simulink model "simulazione_completa"  (R2020a)
settings: Solver=VariableStepAuto  StartTime=0.0  StopTime=1.1*Ts*p  RelTol=1e-3
values from neighbouring files (symbols this model uses):
  A = A_lin_eq    [Ascensione.m]    (also in Sistema.m; f_tilde.m = [-0.0014   -0.0000         0)
  Ad = sysD.a    [Ascensione.m]    (also in Sistema.m)
  B = B_lin_eq(:,1)    [Ascensione.m]    (also in Sistema.m; f_tilde.m = [0.0014)
  Bd = sysD.b    [Ascensione.m]    (also in Sistema.m)
  C = [0 1 0]    [Ascensione.m]    (also in Sistema.m)
  p = 1000    [Pianificazione_senza_vincoli.m]    (also in Pianificazione_vincoli_ingresso.m = p+1; Pianificazione_vincoli_stato.m = ceil(p*1.1); tpr.m = p0*(1-L/T0*z)^(g/(R*L)))
  reg = ss(A+B*K+L*C,-L,-K,0)    [Ascensione.m]    (also in Sistema.m)
  Ts = 0.05    [Ascensione.m]    (also in Sistema.m)
  Vlim = -double(sqrt(2*subs(m,[x1,x2],[x1_eq,x2_eq])*g/rho_bar/Sz/Cz))    [Sistema.m]
  x_0 = [0 0 0].'    [Pianificazione_senza_vincoli.m]
settings Model: Creator=andre  LastModifiedBy=andre
settings OptimizationCC: BlockReduction=off  DefaultParameterBehavior=Inlined  BufferReuse=off

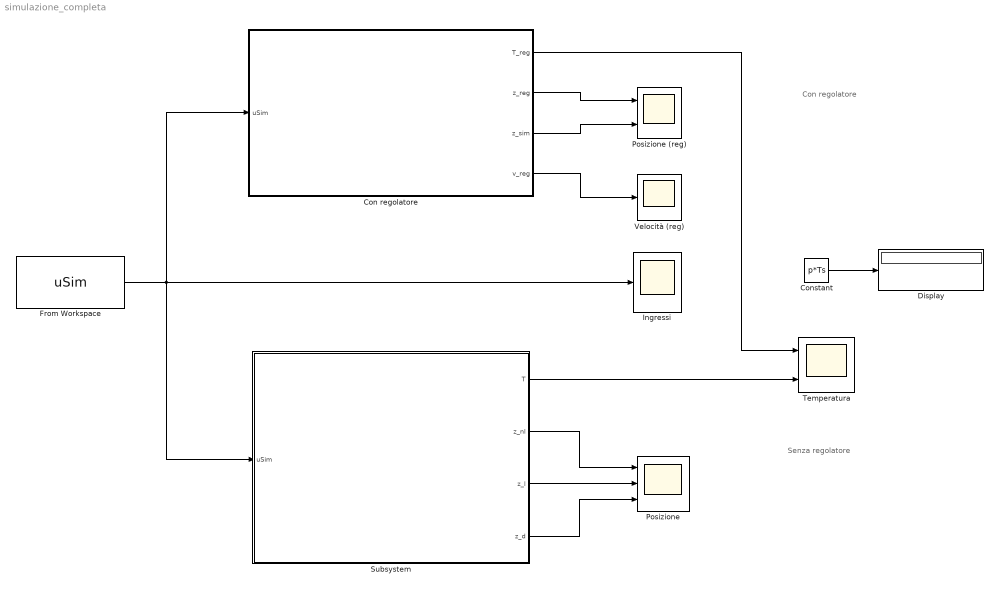
== system simulazione_completa ==
  note: Senza regolatore
  note: Con regolatore
  Con regolatore : Subsystem
  Constant : Constant  Value=p*Ts
  Display : Display
  From Workspace : FromWorkspace  VariableName=uSim  SampleTime=Ts  OutputAfterFinalValue=Holding final value
  Ingressi : Scope
  Posizione : Scope  NumInputPorts=3
  Posizione (reg) : Scope  NumInputPorts=2
  Subsystem : Subsystem
  Temperatura : Scope  NumInputPorts=2
  Velocità (reg) : Scope
  wires:
  From Workspace/1 -> Con regolatore/1(uSim), Subsystem/1(uSim), Ingressi/1
  Con regolatore/2(z_reg) -> Posizione (reg)/1
  Con regolatore/3(z_sim) -> Posizione (reg)/2
  Subsystem/2(z_nl) -> Posizione/1
  Subsystem/3(z_l) -> Posizione/2
  Subsystem/4(z_d) -> Posizione/3
  Con regolatore/4(v_reg) -> Velocità (reg)/1
  Subsystem/1(T) -> Temperatura/2
  Con regolatore/1(T_reg) -> Temperatura/1
  Constant/1 -> Display/1

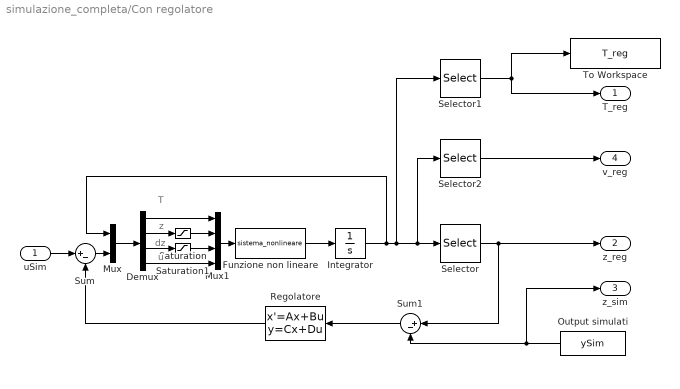
== system simulazione_completa/Con regolatore ==
  note: T
  note: dz
  note: z
  note: u
  uSim : Inport
  Demux : Demux
  Funzione non lineare : MATLABFcn  MATLABFcn=sistema_nonlineare
  Integrator : Integrator  InitialCondition=x_0
  Mux : Mux  Inputs=2
  Mux1 : Mux
  Output simulati : FromWorkspace  VariableName=ySim  OutputAfterFinalValue=Holding final value
  Regolatore : StateSpace  A=reg.a  B=reg.b  C=reg.c  D=reg.d  InitialCondition=[0 0 0]
  Saturation : Saturate  UpperLimit=1000  LowerLimit=-2
  Saturation1 : Saturate  UpperLimit=16  LowerLimit=Vlim
  Selector : Selector  InputPortWidth=3  IndexOptions=Index vector (dialog)  Indices=[2]  OutputSizes=1
  Selector1 : Selector  InputPortWidth=3  IndexOptions=Index vector (dialog)  Indices=[1]  OutputSizes=1
  Selector2 : Selector  InputPortWidth=3  IndexOptions=Index vector (dialog)  Indices=[3]  OutputSizes=1
  Sum : Sum  Inputs=|+-
  Sum1 : Sum  Inputs=|+-
  To Workspace : ToWorkspace  VariableName=T_reg  SampleTime=-1
  T_reg : Outport
  z_reg : Outport  Port=2
  z_sim : Outport  Port=3
  v_reg : Outport  Port=4
  wires:
  uSim/1 -> Sum/1
  Selector1/1 -> T_reg/1, To Workspace/1
  Selector/1 -> z_reg/1, Sum1/1
  Sum1/1 -> Regolatore/1
  Integrator/1 -> Mux/1, Selector1/1, Selector2/1, Selector/1
  Sum/1 -> Mux/2
  Output simulati/1 -> z_sim/1, Sum1/2
  Regolatore/1 -> Sum/2
  Funzione non lineare/1 -> Integrator/1
  Selector2/1 -> v_reg/1
  Demux/1 -> Mux1/1
  Saturation/1 -> Mux1/2
  Demux/2 -> Saturation/1
  Saturation1/1 -> Mux1/3
  Demux/4 -> Mux1/4
  Demux/3 -> Saturation1/1
  Mux/1 -> Demux/1
  Mux1/1 -> Funzione non lineare/1

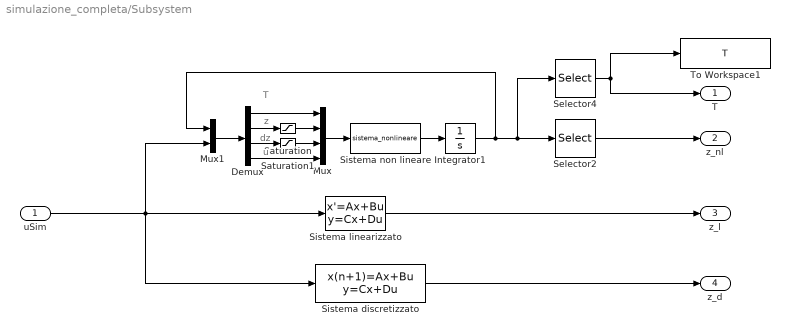
== system simulazione_completa/Subsystem ==
  note: T
  note: z
  note: dz
  note: u
  uSim : Inport
  Demux : Demux
  Integrator1 : Integrator  InitialCondition=x_0
  Mux : Mux
  Mux1 : Mux  Inputs=2
  Saturation : Saturate  UpperLimit=1000  LowerLimit=-2
  Saturation1 : Saturate  UpperLimit=16  LowerLimit=Vlim
  Selector2 : Selector  InputPortWidth=3  IndexOptions=Index vector (dialog)  Indices=[2]  OutputSizes=1
  Selector4 : Selector  InputPortWidth=3  IndexOptions=Index vector (dialog)  Indices=[1]  OutputSizes=1
  Sistema discretizzato : DiscreteStateSpace  A=Ad  B=Bd  C=C  D=0  InitialCondition=x_0  SampleTime=Ts
  Sistema linearizzato : StateSpace  A=A  B=B  C=C  D=0  InitialCondition=x_0
  Sistema non lineare : MATLABFcn  MATLABFcn=sistema_nonlineare
  To Workspace1 : ToWorkspace  VariableName=T  SampleTime=-1
  T : Outport
  z_nl : Outport  Port=2
  z_l : Outport  Port=3
  z_d : Outport  Port=4
  wires:
  Sistema linearizzato/1 -> z_l/1
  Sistema non lineare/1 -> Integrator1/1
  Sistema discretizzato/1 -> z_d/1
  uSim/1 -> Sistema discretizzato/1, Mux1/2, Sistema linearizzato/1
  Selector4/1 -> To Workspace1/1, T/1
  Integrator1/1 -> Mux1/1, Selector4/1, Selector2/1
  Selector2/1 -> z_nl/1
  Demux/2 -> Saturation/1
  Saturation/1 -> Mux/2
  Demux/1 -> Mux/1
  Mux/1 -> Sistema non lineare/1
  Mux1/1 -> Demux/1
  Demux/4 -> Mux/4
  Saturation1/1 -> Mux/3
  Demux/3 -> Saturation1/1
